simulink model "untitled"  (R2017b)
settings: Solver=VariableStepAuto  StartTime=0.0  StopTime=10.0  RelTol=1e-3
settings Model: Creator=DELL-PC  LastModifiedBy=DELL-PC

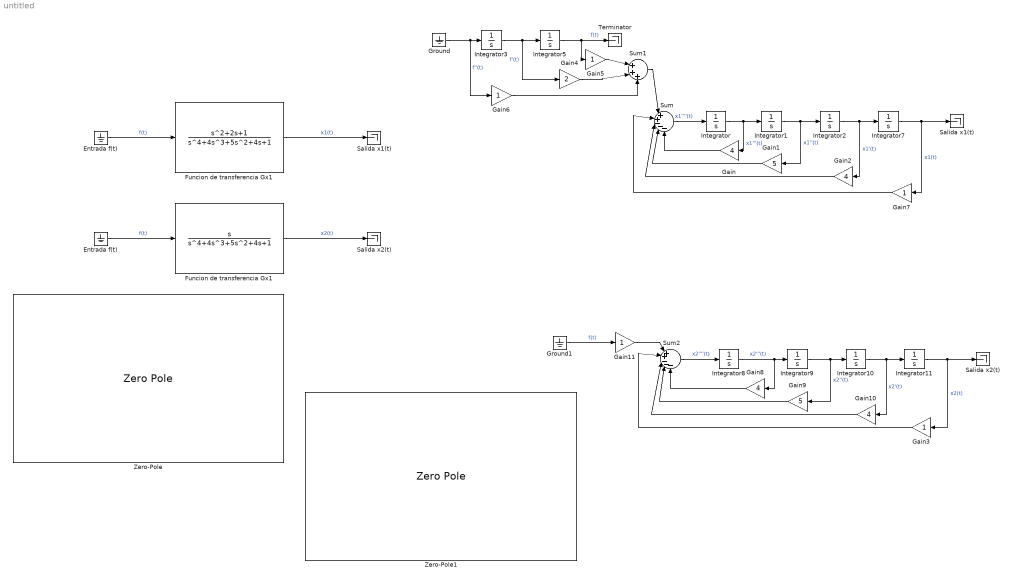
== system untitled ==
  Entrada f(t) : Ground
  "Entrada f(t) " : Ground
  Funcion de transferencia Gx1 : TransferFcn  Numerator=[1 2 1]  Denominator=[1 4 5 4 1]
  "Funcion de transferencia Gx1 " : TransferFcn  Numerator=[0 0 0 1 0]  Denominator=[1 4 5 4 1]
  Gain{,2,8,10} (4 alike) : Gain  Gain=4
  Gain1 : Gain  Gain=5
  Gain{3,5..7,11} (5 alike) : Gain
  Gain4 : Gain  Gain=2
  Gain9 : Gain  Gain=5
  Ground : Ground
  Ground1 : Ground
  Integrator{,1..3,5,7..11} (10 alike) : Integrator
  Salida x1(t) : Terminator
  "Salida x1(t) " : Terminator
  Salida x2(t) : Terminator
  "Salida x2(t) " : Terminator
  Sum : Sum  Inputs=|++---
  Sum1 : Sum  Inputs=|+++
  Sum2 : Sum  Inputs=|++---
  Terminator : Terminator
  Zero-Pole : ZeroPole  Zeros=[-1 -1]  Poles="[(-0.5 -0.8660j)  (-0.5 +0.8660j) -2.6180 -0.3820]"
  Zero-Pole1 : ZeroPole  Zeros=[0]  Poles="[(-0.5 -0.8660j)  (-0.5 +0.8660j) -2.6180 -0.3820]"
  wires:
  Entrada f(t)/1 -> Funcion de transferencia Gx1/1  "f(t)"
  Funcion de transferencia Gx1/1 -> Salida x1(t)/1  "x1(t)"
  "Entrada f(t) "/1 -> "Funcion de transferencia Gx1 "/1  "f(t)"
  "Funcion de transferencia Gx1 "/1 -> Salida x2(t)/1  "x2(t)"
  Sum/1 -> Integrator/1  "x1''''(t)"
  Integrator/1 -> Gain/1, Integrator1/1  "x1'''(t)"
  Integrator1/1 -> Gain1/1, Integrator2/1  "x1''(t)"
  Integrator2/1 -> Gain2/1, Integrator7/1  "x1'(t)"
  Integrator7/1 -> "Salida x1(t) "/1, Gain7/1  "x1(t)"
  Gain/1 -> Sum/5
  Gain1/1 -> Sum/4
  Gain2/1 -> Sum/3
  Gain7/1 -> Sum/2
  Gain8/1 -> Sum2/5
  Sum2/1 -> Integrator8/1  "x2''''(t)"
  Gain9/1 -> Sum2/4
  Integrator8/1 -> Gain8/1, Integrator9/1  "x2'''(t)"
  Integrator9/1 -> Gain9/1, Integrator10/1  "x2''(t)"
  Gain10/1 -> Sum2/3
  Integrator10/1 -> Gain10/1, Integrator11/1  "x2'(t)"
  Integrator11/1 -> Gain3/1, "Salida x2(t) "/1  "x2(t)"
  Gain3/1 -> Sum2/2
  Integrator3/1 -> Gain4/1, Integrator5/1  "f'(t)"
  Integrator5/1 -> Terminator/1, Gain5/1  "f(t)"
  Ground/1 -> Gain6/1, Integrator3/1  "f''(t)"
  Sum1/1 -> Sum/1
  Gain5/1 -> Sum1/1
  Ground1/1 -> Gain11/1  "f(t)"
  Gain11/1 -> Sum2/1
  Gain4/1 -> Sum1/2
  Gain6/1 -> Sum1/3
